simulink model "npc_plant"  (R2022a)
settings: Solver=FixedStepDiscrete  StartTime=0.0  StopTime=Inf  FixedStep=step_size  RelTol=1e-3  EnableMultiTasking=on
undefined symbols (not defined in the file): freq, L, P, step_size, vac_rms, Vdc, Vrms
libraries: spsFirstOrderFilterLib x22, spsSeriesRLCBranchLib x19, spsCurrentMeasurementLib x7, spsMosfetLib x6, spsVoltageMeasurementLib x5, spsACVoltageSourceLib x3, spsIdealSwitchLib x2, spsControlledCurrentSourceLib x1, spsDCVoltageSourceLib x1, spsGroundLib x1, spsPower3phInstantaneousLib x1, spsRMSLib x1
settings Model: DataDictionary=param.sldd  ExtModeTrigDuration=8  Creator=sgcesuser3  LastModifiedBy=sgcesuser3
settings SolverCC: AlgebraicLoopSolver=TrustRegion  AutoInsertRateTranBlk=on
settings OptimizationCC: DefaultUnderspecifiedDataType=single  EnhancedBackFolding=on  PassReuseOutputArgsAs=Individual arguments  MaxStackSize=1024  OptimizeBlockOrder=speed  DifferentSizesBufferReuse=on  OptimizationCustomize=off  DenormalBehavior=FlushToZero  EfficientTunableParamExpr=on
settings DebuggingCC: ParameterTunabilityLossMsg=error  UnconnectedInputMsg=warning  UnconnectedOutputMsg=warning  UnconnectedLineMsg=warning  SFMachineParentedDataDiag=warning
settings HardwareCC: ProdBitPerChar=16  ProdBitPerInt=16  ProdBitPerPointer=32  ProdBitPerSizeT=32  ProdBitPerPtrDiffT=32  ProdLargestAtomicInteger=Integer  ProdLargestAtomicFloat=None  ProdWordSize=16  ProdHWDeviceType=Texas Instruments->C2000
settings ModelReferenceCC: ModelReferenceNumInstancesAllowed=Single
settings SFSimCC: MATLABDynamicMemAlloc=off
settings RTWCC: SystemTargetFile=ert.tlc  HardwareBoard=TI Piccolo F280049C LaunchPad  TemplateMakefile=ert_default_tmf  Toolchain=Texas Instruments Code Composer Studio (C2000)  DLArmComputeVersion=19.05
settings CodeAppCC: ForceParamTrailComments=on  IgnoreCustomStorageClasses=off  OperatorAnnotations=on  SimulinkDataObjDesc=on  SFDataObjDesc=on  InsertBlockDesc=on
settings ERTTargetCC: CodeReplacementLibrary=TI C28x  ExtModeTransport=3  ExtModeStaticAllocSize=5000

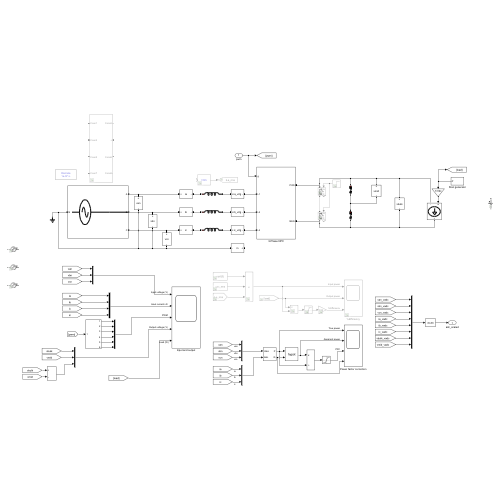
[thumbnail: Simulink's stored preview of the top-level diagram]
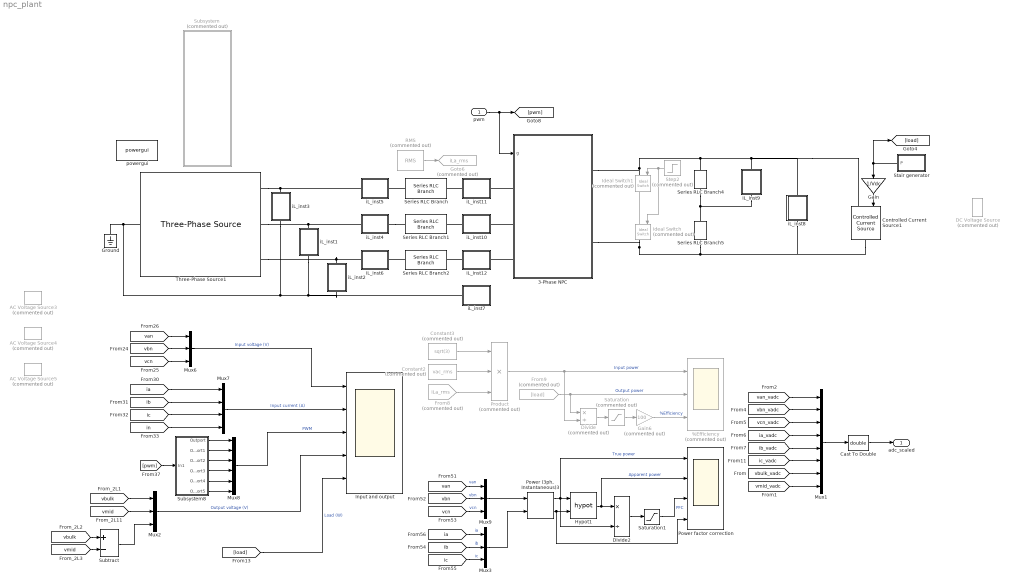
== system npc_plant ==
  pwm : Inport
  %Efficiency : Scope  Commented=on  NumInputPorts=3
  3-Phase NPC : Subsystem
  AC Voltage Source3 : spsACVoltageSourceLib/AC Voltage Source  Commented=on  Amplitude=325  Phase=0  Frequency=50  SampleTime=-1  Measurements=None  BusType=swing  Pref=10e3  Qref=0  Qmin=-inf  Qmax=+inf
  AC Voltage Source4 : spsACVoltageSourceLib/AC Voltage Source  Commented=on  Amplitude=325  Phase=0  Frequency=50  SampleTime=-1  Measurements=None  BusType=swing  Pref=10e3  Qref=0  Qmin=-inf  Qmax=+inf
  AC Voltage Source5 : spsACVoltageSourceLib/AC Voltage Source  Commented=on  Amplitude=325  Phase=0  Frequency=50  SampleTime=-1  Measurements=None  BusType=swing  Pref=10e3  Qref=0  Qmin=-inf  Qmax=+inf
  Cast To Double : DataTypeConversion  OutDataTypeStr=double  SaturateOnIntegerOverflow=off  RndMeth=Floor
  Constant2 : Constant  Commented=on  Value=vac_rms
  Constant3 : Constant  Commented=on  Value=sqrt(3)
  Controlled Current Source1 : spsControlledCurrentSourceLib/Controlled Current Source  Initialize=on  Source_Type=DC  Amplitude=0  Phase=0  Frequency=0  Measurements=None
  DC Voltage Source : spsDCVoltageSourceLib/DC Voltage Source  Commented=on  Amplitude=Vdc  Measurements=None
  Divide : Product  Commented=on  Inputs=*/
  Divide2 : Product  Inputs=*/
  From8 : From  Commented=on  GotoTag=iLa_rms  TagVisibility=global
  From9 : From  Commented=on  GotoTag=load
  Gain : Gain  Gain=1/Vdc
  Gain6 : Gain  Commented=on  Gain=100
  Goto6 : Goto  Commented=on  GotoTag=iLa_rms  TagVisibility=global
  Ground : spsGroundLib/Ground  LConnTagsString=a
  Hypot1 : Math  Operator=hypot
  Ideal Switch : spsIdealSwitchLib/Ideal Switch  Commented=on  Ron=5  Lon=0  IC=0  Rs=1e5  Cs=inf  Measurements=on
  Ideal Switch1 : spsIdealSwitchLib/Ideal Switch  Commented=on  Ron=4  Lon=0  IC=0  Rs=1e5  Cs=inf  Measurements=on
  Input and output : Scope  NumInputPorts=5
  Mux1 : Mux  Inputs=8
  Mux{2..3,6,9} (4 alike) : Mux  Inputs=3
  Mux7 : Mux
  Mux8 : Mux  Inputs=6
  "Power (3ph, Instantaneous)3" : spsPower3phInstantaneousLib/Power (3ph, Instantaneous)
  Power factor correction : Scope  NumInputPorts=4
  Product : Product  Commented=on  Inputs=3
  RMS : spsRMSLib/RMS  Commented=on  TrueRMS=on  Freq=freq  RMSInit=freq*2  Ts=step_size
  Saturation : Saturate  Commented=on  UpperLimit=1  LowerLimit=0
  Saturation1 : Saturate  UpperLimit=1  LowerLimit=0
  Series RLC Branch : spsSeriesRLCBranchLib/Series RLC Branch  LConnTagsString=__new0  RConnTagsString=__new0  BranchType=L  Resistance=1  Inductance=L  SetiL0=off  InitialCurrent=0  Capacitance=1e-6  Setx0=off  InitialVoltage=0  Measurements=None
  Series RLC Branch1 : spsSeriesRLCBranchLib/Series RLC Branch  LConnTagsString=__new0  RConnTagsString=__new0  BranchType=L  Resistance=1  Inductance=L  SetiL0=off  InitialCurrent=0  Capacitance=1e-6  Setx0=off  InitialVoltage=0  Measurements=None
  Series RLC Branch2 : spsSeriesRLCBranchLib/Series RLC Branch  LConnTagsString=__new0  RConnTagsString=__new0  BranchType=L  Resistance=1  Inductance=L  SetiL0=off  InitialCurrent=0  Capacitance=1e-6  Setx0=off  InitialVoltage=0  Measurements=None
  Series RLC Branch4 : spsSeriesRLCBranchLib/Series RLC Branch  LConnTagsString=__new0  RConnTagsString=__new0  BranchType=RC  Resistance=1e-3  Inductance=182e-6  SetiL0=off  InitialCurrent=0  Capacitance=2160e-6  Setx0=on  InitialVoltage=Vrms*sqrt(2)*sqrt(3)/2  Measurements=None
  Series RLC Branch5 : spsSeriesRLCBranchLib/Series RLC Branch  LConnTagsString=__new0  RConnTagsString=__new0  BranchType=RC  Resistance=1e-3  Inductance=182e-6  SetiL0=off  InitialCurrent=0  Capacitance=2160e-6  Setx0=on  InitialVoltage=Vrms*sqrt(2)*sqrt(3)/2  Measurements=None
  Stair generator : Subsystem
  Step2 : Step  Commented=on  Time=10  SampleTime=0
  Subsystem : Subsystem  Commented=on
  Subsystem8 : Subsystem
  Subtract : Sum  Inputs=+-
  Three-Phase Source1 : spsThreePhaseSourceLib/Three-Phase Source  InternalConnection=Yn  VoltagePhases=off  Voltage=Vrms*sqrt(3)  PhaseAngle=0  Voltage_phases=[25e3 25e3 25e3]/sqrt(3)  PhaseAngles_phases=[0 -120 +120]  Frequency=50  NonIdealSource=off  SpecifyImpedance=off  Resistance=0.8929  Inductance=16.58e-3  ShortCircuitLevel=100e6  BaseVoltage=25e3  XRratio=7  BusType=swing  Pref=10e3  Qref=0  Prefabc=[10e3, 10e3, 10e3]  Qrefabc=[0, 0, 0]  Qmin=-inf  Qmax=inf
  iL_inst1 : Subsystem
      mask Display:
      | disp('vbn')
      | port_label('Lconn',1,'+')
      | port_label('Rconn',1,'-')
  iL_inst10 : Subsystem
      mask Display:
      | disp('ib_v2g')
      | port_label('Lconn',1,'+')
      | port_label('Rconn',1,'-')
  iL_inst11 : Subsystem
      mask Display:
      | disp('ia_v2g')
      | port_label('Lconn',1,'+')
      | port_label('Rconn',1,'-')
  iL_inst12 : Subsystem
      mask Display:
      | disp('ic_v2g')
      | port_label('Lconn',1,'+')
      | port_label('Rconn',1,'-')
  iL_inst2 : Subsystem
      mask Display:
      | disp('vcn')
      | port_label('Lconn',1,'+')
      | port_label('Rconn',1,'-')
  iL_inst3 : Subsystem
      mask Display:
      | disp('van')
      | port_label('Lconn',1,'+')
      | port_label('Rconn',1,'-')
  iL_inst4 : Subsystem
      mask Display:
      | disp('ib')
      | port_label('Lconn',1,'+')
      | port_label('Rconn',1,'-')
  iL_inst5 : Subsystem
      mask Display:
      | disp('ia')
      | port_label('Lconn',1,'+')
      | port_label('Rconn',1,'-')
  iL_inst6 : Subsystem
      mask Display:
      | disp('ic')
      | port_label('Lconn',1,'+')
      | port_label('Rconn',1,'-')
  iL_inst7 : Subsystem
      mask Display:
      | disp('in')
      | port_label('Lconn',1,'+')
      | port_label('Rconn',1,'-')
  iL_inst8 : Subsystem
      mask Display:
      | disp('vbulk')
      | port_label('Lconn',1,'+')
      | port_label('Rconn',1,'-')
  iL_inst9 : Subsystem
      mask Display:
      | disp('vmid')
      | port_label('Lconn',1,'+')
      | port_label('Rconn',1,'-')
  powergui : spspowerguiLib/powergui  Priority=1  SimulationMode=Discrete  SampleTime=step_size  frequency=60  Iterations=50  frequencyindice=0  Pbase=100e6  ErrMax=1e-4  UnitsV=kV  UnitsW=MW  buscounter=0  FunctionMessages=off  echomessages=off  EnableUseOfTLC=off  CurrentSourceSwitches=off  DisableSnubberDevices=off  DisableRonSwitches=off  DisableVfSwitches=off  DisplayEquations=off  AutomaticDiscreteSolvers=off  SolverType=Tustin/Backward Euler (TBE)  Interpol=off  ExternalGateDelay=off  methode=off  Ts=100  x0status=blocks  SPID=on  SwTol=0  HookPort=off  NonlinearTolerance=1e-4  nMaxIteration=100  ContinueOnMaxIteration=off  RestoreLinks=warning  ResistiveCurrentMeasurement=off  Frange=[0:2:500]  Ylog=off  Xlog=on  ShowGrid=off  save=off  variable=ZData  structure=iLa  ZoomFFT=off  StartTime=0.12  cycles=3  DisplayStyle=2  fundamental=50  FreqAxis=on  MaxFrequency=50*41  frequencyindicesteady=1  RmsSteady=1  display=off
  adc_scaled : Outport
  wires:
  Mux1/1 -> Cast To Double/1
  Cast To Double/1 -> adc_scaled/1
  [van_vadc] -> Mux1/1
  [vbn_vadc] -> Mux1/2
  [vcn_vadc] -> Mux1/3
  [ia_vadc] -> Mux1/4
  [ic_vadc] -> Mux1/6
  [vbulk_vadc] -> Mux1/7
  [vmid_vadc] -> Mux1/8
  pwm/1 -> 3-Phase NPC/1(g), [pwm]
  Mux2/1 -> Input and output/4  "Output voltage (V)"
  [vcn] -> Mux6/3
  [van] -> Mux6/1
  [vbn] -> Mux6/2
  Mux6/1 -> Input and output/1  "Input voltage (V)"
  Mux7/1 -> Input and output/2  "Input current (A)"
  [ia] -> Mux7/1
  [ib] -> Mux7/2
  [ic] -> Mux7/3
  [pwm] -> Subsystem8/1(In1)
  Subsystem8/1(Outport) -> Mux8/1
  Subsystem8/2(Outport1) -> Mux8/2
  Subsystem8/3(Outport2) -> Mux8/3
  Subsystem8/5(Outport4) -> Mux8/5
  Subsystem8/4(Outport3) -> Mux8/4
  Subsystem8/6(Outport5) -> Mux8/6
  Mux8/1 -> Input and output/3  "PWM"
  [in] -> Mux7/4
  Step2/1 -> Ideal Switch/1, Ideal Switch1/1
  [load] -> Input and output/5  "Load (W)"
  [vmid] -> Subtract/2
  [vbulk] -> Subtract/1
  Subtract/1 -> Mux2/3
  [vmid] -> Mux2/2
  [vbulk] -> Mux2/1
  Constant3/1 -> Product/1
  Constant2/1 -> Product/2
  From8/1 -> Product/3
  Gain6/1 -> %Efficiency/3  "%Efficiency"
  Saturation/1 -> Gain6/1
  Product/1 -> Divide/2, %Efficiency/1  "Input power"
  From9/1 -> %Efficiency/2, Divide/1  "Output power"
  Divide/1 -> Saturation/1
  RMS/1 -> Goto6/1
  Saturation1/1 -> Power factor correction/3  "PFC"
  "Power (3ph, Instantaneous)3"/2 -> Power factor correction/4, Hypot1/2
  Mux9/1 -> "Power (3ph, Instantaneous)3"/1
  Mux3/1 -> "Power (3ph, Instantaneous)3"/2
  Hypot1/1 -> Divide2/1, Power factor correction/2  "Apparent power"
  "Power (3ph, Instantaneous)3"/1 -> Hypot1/1, Power factor correction/1, Divide2/2  "True power"
  Divide2/1 -> Saturation1/1
  [ic] -> Mux3/3  "ic"
  [vbn] -> Mux9/2  "vbn"
  [ib] -> Mux3/2  "ib"
  [ia] -> Mux3/1  "ia"
  [van] -> Mux9/1  "van"
  [vcn] -> Mux9/3  "vcn"
  [ib_vadc] -> Mux1/5
  Stair generator/1(P) -> Gain/1, [load]
  Gain/1 -> Controlled Current Source1/1
  connections:
  iL_inst5/LConn1 -- Three-Phase Source1/RConn1 -- iL_inst3/LConn1
  3-Phase NPC/RConn2 -- Ideal Switch/RConn1 -- Controlled Current Source1/RConn1 -- iL_inst8/RConn1 -- Series RLC Branch5/RConn1
  iL_inst4/LConn1 -- Three-Phase Source1/RConn2 -- iL_inst1/LConn1
  3-Phase NPC/LConn1 -- iL_inst11/RConn1
  iL_inst4/RConn1 -- Series RLC Branch1/LConn1
  3-Phase NPC/LConn2 -- iL_inst10/RConn1
  3-Phase NPC/LConn3 -- iL_inst12/RConn1
  Series RLC Branch/LConn1 -- iL_inst5/RConn1
  iL_inst2/LConn1 -- iL_inst6/LConn1 -- Three-Phase Source1/RConn3
  Series RLC Branch2/LConn1 -- iL_inst6/RConn1
  3-Phase NPC/RConn1 -- Ideal Switch1/LConn1 -- Controlled Current Source1/LConn1 -- iL_inst8/LConn1 -- iL_inst9/LConn1 -- Series RLC Branch4/LConn1
  iL_inst11/LConn1 -- Series RLC Branch/RConn1
  iL_inst10/LConn1 -- Series RLC Branch1/RConn1
  iL_inst12/LConn1 -- Series RLC Branch2/RConn1
  Ground/LConn1 -- Three-Phase Source1/LConn1 -- iL_inst3/RConn1 -- iL_inst1/RConn1 -- iL_inst2/RConn1 -- iL_inst7/RConn1
  Series RLC Branch5/LConn1 -- iL_inst9/RConn1 -- Series RLC Branch4/RConn1
  Ideal Switch/LConn1 -- Ideal Switch1/RConn1

== system npc_plant/3-Phase NPC ==
  g : Inport
  NPC_A : Subsystem
      settings: PortSchema="{\"entries\":[{\"content\":{\"sides\":[{\"content\":{\"connectorIds\":[\"LConn1\",\"LConn2\",\"LConn3\",\"In1\"]},\"type\":\"ConnectorPlacement.EquallySpacedRectSide\",\"uuid\":\"185b644c-5e86-499b-a0c5-6bf9ed4f6992\"},{\"content\":{\"connectorIds\":[\"RConn1\",\"RConn2\"],\"side\":\"RIGHT\"},\"type\":\"ConnectorPlacement.EquallySpacedRectSide\",\"uuid\":\"b556d60a-a111-4d52-8667-7aa86b258dfe\"},{\"content\":{\"connectorIds\":[],\"side\":\"TOP\"},\"type\":\"ConnectorPlacement.EquallySpacedRectSide\",\"uuid\":\"a387e194-6dea-4371-ac8c-2c0bb28b101b\"},{\"content\":{\"connectorIds\":[],\"side\":\"HIDDEN\"},\"type\":\"ConnectorPlacement.EquallySpacedRectSide\",\"uuid\":\"89f90e44-d209-472d-9123-cabb2f2076c2\"}]},\"type\":\"ConnectorPlacement.EquallySpacedConnector\",\"uuid\":\"47575041-459b-4ece-9f52-08593f67c377\"}],\"packageUris\":[\"http://schema.mathworks.com/mf0/Connector/R2020b\"],\"version\":\"1.0\"}"
  Series RLC Branch : spsSeriesRLCBranchLib/Series RLC Branch  LConnTagsString=__new0  RConnTagsString=__new0  BranchType=R  Resistance=1e-3  Inductance=1e-3  SetiL0=off  InitialCurrent=0  Capacitance=1e-6  Setx0=off  InitialVoltage=0  Measurements=None
  Series RLC Branch1 : spsSeriesRLCBranchLib/Series RLC Branch  LConnTagsString=__new0  RConnTagsString=__new0  BranchType=R  Resistance=1e-3  Inductance=1e-3  SetiL0=off  InitialCurrent=0  Capacitance=1e-6  Setx0=off  InitialVoltage=0  Measurements=None
  Series RLC Branch2 : spsSeriesRLCBranchLib/Series RLC Branch  LConnTagsString=__new0  RConnTagsString=__new0  BranchType=R  Resistance=1e-3  Inductance=1e-3  SetiL0=off  InitialCurrent=0  Capacitance=1e-6  Setx0=off  InitialVoltage=0  Measurements=None
  L1 : PMIOPort  Side=Left
  L2 : PMIOPort  Port=2  Side=Left
  L3 : PMIOPort  Port=3  Side=Left
  POS : PMIOPort  Port=4  Side=Right
  NEG : PMIOPort  Port=5  Side=Right
  wires:
  g/1 -> NPC_A/1(g)
  connections:
  Series RLC Branch/LConn1 -- L1/RConn1
  Series RLC Branch1/LConn1 -- L2/RConn1
  Series RLC Branch2/LConn1 -- L3/RConn1
  Series RLC Branch/RConn1 -- NPC_A/LConn1
  Series RLC Branch1/RConn1 -- NPC_A/LConn2
  Series RLC Branch2/RConn1 -- NPC_A/LConn3
  NPC_A/RConn1 -- POS/RConn1
  NEG/RConn1 -- NPC_A/RConn2

== system npc_plant/Stair generator ==
  1% : Subsystem  TreatAsAtomicUnit=on
  10% : Subsystem  TreatAsAtomicUnit=on
  100% : Subsystem  TreatAsAtomicUnit=on
  25% : Subsystem  TreatAsAtomicUnit=on
  50% : Subsystem  TreatAsAtomicUnit=on
  Digital Clock : DigitalClock  SampleTime=-1
  If : If  IfExpression=u1 > 0.7  ElseIfExpressions=u1 > 0.6, u1 > 0.5, u1 > 0.4, u1 >= 0
  Merge : Merge  Inputs=5
  P : Outport
  wires:
  Digital Clock/1 -> If/1
  If/2 -> 50%/Action
  If/4 -> 10%/Action
  If/5 -> 1%/Action
  Merge/1 -> P/1
  25%/1(Out1) -> Merge/3
  100%/1(Out1) -> Merge/1
  50%/1(Out1) -> Merge/2
  10%/1(Out1) -> Merge/4
  1%/1(Out1) -> Merge/5
  If/1 -> 100%/Action
  If/3 -> 25%/Action

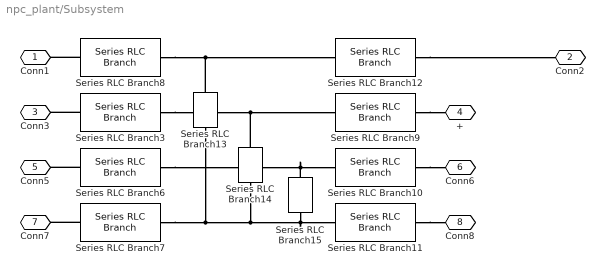
== system npc_plant/Subsystem ==
  Series RLC Branch{3,6..12} (8 alike) : spsSeriesRLCBranchLib/Series RLC Branch  LConnTagsString=__new0  RConnTagsString=__new0  BranchType=L  Resistance=1  Inductance=1.4e-3  SetiL0=off  InitialCurrent=0  Capacitance=1e-6  Setx0=off  InitialVoltage=0  Measurements=None
  Series RLC Branch13 : spsSeriesRLCBranchLib/Series RLC Branch  LConnTagsString=__new0  RConnTagsString=__new0  BranchType=C  Resistance=1  Inductance=182e-6  SetiL0=off  InitialCurrent=0  Capacitance=2.2e-6  Setx0=on  InitialVoltage=0  Measurements=None
  Series RLC Branch14 : spsSeriesRLCBranchLib/Series RLC Branch  LConnTagsString=__new0  RConnTagsString=__new0  BranchType=C  Resistance=1  Inductance=182e-6  SetiL0=off  InitialCurrent=0  Capacitance=2.2e-6  Setx0=on  InitialVoltage=0  Measurements=None
  Series RLC Branch15 : spsSeriesRLCBranchLib/Series RLC Branch  LConnTagsString=__new0  RConnTagsString=__new0  BranchType=C  Resistance=1  Inductance=182e-6  SetiL0=off  InitialCurrent=0  Capacitance=2.2e-6  Setx0=on  InitialVoltage=0  Measurements=None
  Conn1 : PMIOPort  Side=Left
  Conn2 : PMIOPort  Port=2  Side=Right
  Conn3 : PMIOPort  Port=3  Side=Left
  + : PMIOPort  Port=4  Side=Right
  Conn5 : PMIOPort  Port=5  Side=Left
  Conn6 : PMIOPort  Port=6  Side=Right
  Conn7 : PMIOPort  Port=7  Side=Left
  Conn8 : PMIOPort  Port=8  Side=Right
  connections:
  Series RLC Branch9/RConn1 -- +/RConn1
  Series RLC Branch7/RConn1 -- Series RLC Branch13/RConn1 -- Series RLC Branch14/RConn1 -- Series RLC Branch15/RConn1 -- Series RLC Branch11/LConn1
  Series RLC Branch8/RConn1 -- Series RLC Branch13/LConn1 -- Series RLC Branch12/LConn1
  Series RLC Branch6/LConn1 -- Conn5/RConn1
  Series RLC Branch7/LConn1 -- Conn7/RConn1
  Series RLC Branch6/RConn1 -- Series RLC Branch15/LConn1 -- Series RLC Branch10/LConn1
  Series RLC Branch3/RConn1 -- Series RLC Branch14/LConn1 -- Series RLC Branch9/LConn1
  Series RLC Branch12/RConn1 -- Conn2/RConn1
  Series RLC Branch11/RConn1 -- Conn8/RConn1
  Series RLC Branch10/RConn1 -- Conn6/RConn1
  Series RLC Branch3/LConn1 -- Conn3/RConn1
  Series RLC Branch8/LConn1 -- Conn1/RConn1

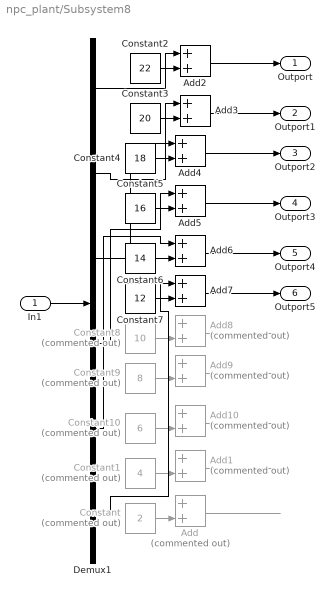
== system npc_plant/Subsystem8 ==
  In1 : Inport
  Add{,1,8..10} (5 alike) : Sum  Commented=on
  Add{2..7} (6 alike) : Sum
  Constant : Constant  Commented=on  Value=2
  Constant1 : Constant  Commented=on  Value=4
  Constant10 : Constant  Commented=on  Value=6
  Constant2 : Constant  Value=22
  Constant3 : Constant  Value=20
  Constant4 : Constant  Value=18
  Constant5 : Constant  Value=16
  Constant6 : Constant  Value=14
  Constant7 : Constant  Value=12
  Constant8 : Constant  Commented=on  Value=10
  Constant9 : Constant  Commented=on  Value=8
  Demux1 : Demux  Outputs=6
  Outport : Outport
  Outport1 : Outport  Port=2
  Outport2 : Outport  Port=3
  Outport3 : Outport  Port=4
  Outport4 : Outport  Port=5
  Outport5 : Outport  Port=6
  wires:
  ? -> Add/1
  In1/1 -> Demux1/1
  Constant/1 -> Add/2
  ? -> Add1/1
  Constant1/1 -> Add1/2
  Constant2/1 -> Add2/2
  Demux1/1 -> Add2/1
  Demux1/2 -> Add3/1
  Constant3/1 -> Add3/2
  Constant4/1 -> Add4/2
  Demux1/3 -> Add4/1
  Constant5/1 -> Add5/2
  Constant6/1 -> Add6/2
  Constant7/1 -> Add7/2
  Constant8/1 -> Add8/2
  Constant9/1 -> Add9/2
  Constant10/1 -> Add10/2
  Demux1/4 -> Add5/1
  Demux1/5 -> Add6/1
  Demux1/6 -> Add7/1
  ? -> Add8/1
  ? -> Add9/1
  ? -> Add10/1
  Add5/1 -> Outport3/1
  Add4/1 -> Outport2/1
  Add3/1 -> Outport1/1
  Add2/1 -> Outport/1
  Add6/1 -> Outport4/1
  Add7/1 -> Outport5/1
  Add8/1 -> ?
  Add9/1 -> ?
  Add10/1 -> ?
  Add1/1 -> ?
  Add/1 -> ?
  ? -> ?

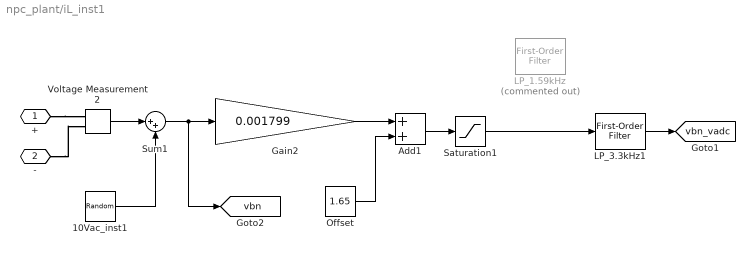
== system npc_plant/iL_inst1 ==
  10Vac_inst1 : RandomNumber  Variance=0
  Add1 : Sum
  Gain2 : Gain  Gain=0.001799
  LP_1.59kHz : spsFirstOrderFilterLib/First-Order Filter  Commented=on  FilterType=Lowpass  Tc=10e3*10e-9  Ts=step_size  Initialize=on  Vac_Init=[0, 0, 60]  Vdc_Init=0  PlotResponse=off  FreqRange="[0,  200,  1]"
  LP_3.3kHz1 : spsFirstOrderFilterLib/First-Order Filter  FilterType=Lowpass  Tc=47e-6  Ts=step_size  Initialize=on  Vac_Init=[0, 0, 60]  Vdc_Init=0  PlotResponse=off  FreqRange="[0,  200,  1]"
  Offset : Constant  Value=1.65  OutDataTypeStr=single
  Saturation1 : Saturate  UpperLimit=3.3  LowerLimit=0
  Sum1 : Sum  Inputs=|++
  Voltage Measurement2 : spsVoltageMeasurementLib/Voltage Measurement  PhasorSimulation=off  OutputType=Complex  PSBequivalent=0
  + : PMIOPort  Side=Left
  - : PMIOPort  Port=2  Side=Right
  tag scope: vbn=global, vbn_vadc=global
  wires:
  Sum1/1 -> [vbn], Gain2/1
  Offset/1 -> Add1/2
  Add1/1 -> Saturation1/1
  Gain2/1 -> Add1/1
  10Vac_inst1/1 -> Sum1/2
  Voltage Measurement2/1 -> Sum1/1
  Saturation1/1 -> LP_3.3kHz1/1
  LP_3.3kHz1/1 -> [vbn_vadc]
  connections:
  -/RConn1 -- Voltage Measurement2/LConn2
  +/RConn1 -- Voltage Measurement2/LConn1

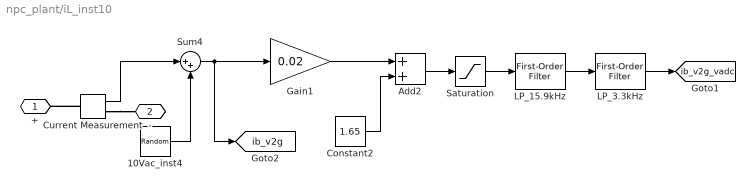
== system npc_plant/iL_inst10 ==
  10Vac_inst4 : RandomNumber  Variance=0
  Add2 : Sum
  Constant2 : Constant  Value=1.65  OutDataTypeStr=single
  Current Measurement : spsCurrentMeasurementLib/Current Measurement  PhasorSimulation=off  OutputType=Complex  PSBequivalent=0
  Gain1 : Gain  Gain=0.02
  LP_15.9kHz : spsFirstOrderFilterLib/First-Order Filter  FilterType=Lowpass  Tc=10e-6  Ts=step_size  Initialize=on  Vac_Init=[0, 0, 60]  Vdc_Init=0  PlotResponse=off  FreqRange="[0,  200,  1]"
  LP_3.3kHz : spsFirstOrderFilterLib/First-Order Filter  FilterType=Lowpass  Tc=47e-6  Ts=step_size  Initialize=on  Vac_Init=[0, 0, 60]  Vdc_Init=0  PlotResponse=off  FreqRange="[0,  200,  1]"
  Saturation : Saturate  UpperLimit=3.3  LowerLimit=0
  Sum4 : Sum  Inputs=|++
  + : PMIOPort  Side=Left
  - : PMIOPort  Port=2  Side=Right
  tag scope: ib_v2g=global, ib_v2g_vadc=global
  wires:
  10Vac_inst4/1 -> Sum4/2
  Current Measurement/1 -> Sum4/1
  Add2/1 -> Saturation/1
  Sum4/1 -> Gain1/1, [ib_v2g]
  Gain1/1 -> Add2/1
  Constant2/1 -> Add2/2
  LP_3.3kHz/1 -> [ib_v2g_vadc]
  LP_15.9kHz/1 -> LP_3.3kHz/1
  Saturation/1 -> LP_15.9kHz/1
  connections:
  Current Measurement/RConn1 -- -/RConn1
  Current Measurement/LConn1 -- +/RConn1

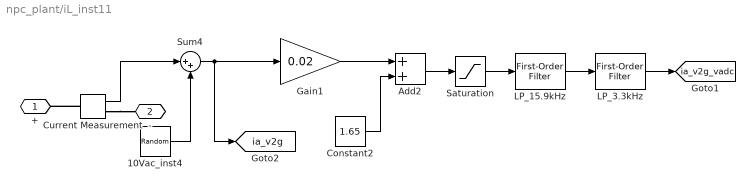
== system npc_plant/iL_inst11 ==
  10Vac_inst4 : RandomNumber  Variance=0
  Add2 : Sum
  Constant2 : Constant  Value=1.65  OutDataTypeStr=single
  Current Measurement : spsCurrentMeasurementLib/Current Measurement  PhasorSimulation=off  OutputType=Complex  PSBequivalent=0
  Gain1 : Gain  Gain=0.02
  LP_15.9kHz : spsFirstOrderFilterLib/First-Order Filter  FilterType=Lowpass  Tc=10e-6  Ts=step_size  Initialize=on  Vac_Init=[0, 0, 60]  Vdc_Init=0  PlotResponse=off  FreqRange="[0,  200,  1]"
  LP_3.3kHz : spsFirstOrderFilterLib/First-Order Filter  FilterType=Lowpass  Tc=47e-6  Ts=step_size  Initialize=on  Vac_Init=[0, 0, 60]  Vdc_Init=0  PlotResponse=off  FreqRange="[0,  200,  1]"
  Saturation : Saturate  UpperLimit=3.3  LowerLimit=0
  Sum4 : Sum  Inputs=|++
  + : PMIOPort  Side=Left
  - : PMIOPort  Port=2  Side=Right
  tag scope: ia_v2g=global, ia_v2g_vadc=global
  wires:
  Saturation/1 -> LP_15.9kHz/1
  LP_15.9kHz/1 -> LP_3.3kHz/1
  LP_3.3kHz/1 -> [ia_v2g_vadc]
  Constant2/1 -> Add2/2
  Gain1/1 -> Add2/1
  Sum4/1 -> [ia_v2g], Gain1/1
  Add2/1 -> Saturation/1
  Current Measurement/1 -> Sum4/1
  10Vac_inst4/1 -> Sum4/2
  connections:
  Current Measurement/LConn1 -- +/RConn1
  Current Measurement/RConn1 -- -/RConn1

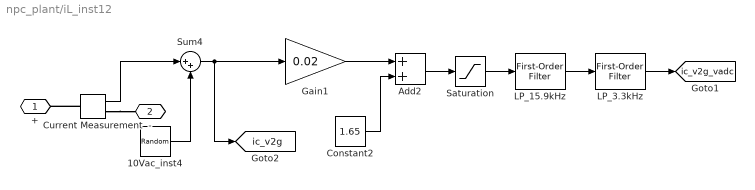
== system npc_plant/iL_inst12 ==
  10Vac_inst4 : RandomNumber  Variance=0
  Add2 : Sum
  Constant2 : Constant  Value=1.65  OutDataTypeStr=single
  Current Measurement : spsCurrentMeasurementLib/Current Measurement  PhasorSimulation=off  OutputType=Complex  PSBequivalent=0
  Gain1 : Gain  Gain=0.02
  LP_15.9kHz : spsFirstOrderFilterLib/First-Order Filter  FilterType=Lowpass  Tc=10e-6  Ts=step_size  Initialize=on  Vac_Init=[0, 0, 60]  Vdc_Init=0  PlotResponse=off  FreqRange="[0,  200,  1]"
  LP_3.3kHz : spsFirstOrderFilterLib/First-Order Filter  FilterType=Lowpass  Tc=47e-6  Ts=step_size  Initialize=on  Vac_Init=[0, 0, 60]  Vdc_Init=0  PlotResponse=off  FreqRange="[0,  200,  1]"
  Saturation : Saturate  UpperLimit=3.3  LowerLimit=0
  Sum4 : Sum  Inputs=|++
  + : PMIOPort  Side=Left
  - : PMIOPort  Port=2  Side=Right
  tag scope: ic_v2g=global, ic_v2g_vadc=global
  wires:
  10Vac_inst4/1 -> Sum4/2
  Current Measurement/1 -> Sum4/1
  Add2/1 -> Saturation/1
  Sum4/1 -> Gain1/1, [ic_v2g]
  Gain1/1 -> Add2/1
  Constant2/1 -> Add2/2
  LP_3.3kHz/1 -> [ic_v2g_vadc]
  LP_15.9kHz/1 -> LP_3.3kHz/1
  Saturation/1 -> LP_15.9kHz/1
  connections:
  Current Measurement/RConn1 -- -/RConn1
  Current Measurement/LConn1 -- +/RConn1

== system npc_plant/iL_inst2 ==
  10Vac_inst1 : RandomNumber  Variance=0
  Add1 : Sum
  Gain2 : Gain  Gain=0.001799
  LP_1.59kHz : spsFirstOrderFilterLib/First-Order Filter  Commented=on  FilterType=Lowpass  Tc=10e3*10e-9  Ts=step_size  Initialize=on  Vac_Init=[0, 0, 60]  Vdc_Init=0  PlotResponse=off  FreqRange="[0,  200,  1]"
  LP_3.3kHz1 : spsFirstOrderFilterLib/First-Order Filter  FilterType=Lowpass  Tc=47e-6  Ts=step_size  Initialize=on  Vac_Init=[0, 0, 60]  Vdc_Init=0  PlotResponse=off  FreqRange="[0,  200,  1]"
  Offset : Constant  Value=1.65  OutDataTypeStr=single
  Saturation1 : Saturate  UpperLimit=3.3  LowerLimit=0
  Sum1 : Sum  Inputs=|++
  Voltage Measurement2 : spsVoltageMeasurementLib/Voltage Measurement  PhasorSimulation=off  OutputType=Complex  PSBequivalent=0
  + : PMIOPort  Side=Left
  - : PMIOPort  Port=2  Side=Right
  tag scope: vcn=global, vcn_vadc=global
  wires:
  LP_3.3kHz1/1 -> [vcn_vadc]
  Saturation1/1 -> LP_3.3kHz1/1
  Voltage Measurement2/1 -> Sum1/1
  10Vac_inst1/1 -> Sum1/2
  Gain2/1 -> Add1/1
  Add1/1 -> Saturation1/1
  Offset/1 -> Add1/2
  Sum1/1 -> Gain2/1, [vcn]
  connections:
  +/RConn1 -- Voltage Measurement2/LConn1
  -/RConn1 -- Voltage Measurement2/LConn2

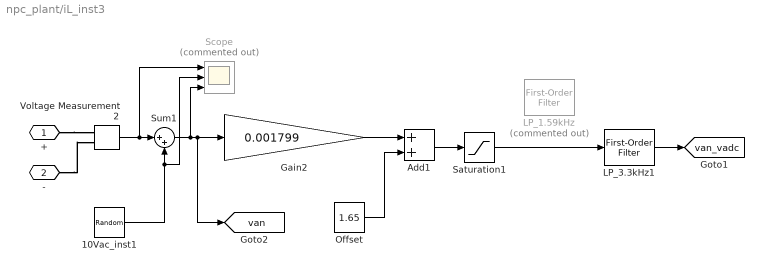
== system npc_plant/iL_inst3 ==
  10Vac_inst1 : RandomNumber  Variance=0
  Add1 : Sum
  Gain2 : Gain  Gain=0.001799
  LP_1.59kHz : spsFirstOrderFilterLib/First-Order Filter  Commented=on  FilterType=Lowpass  Tc=10e3*10e-9  Ts=step_size  Initialize=on  Vac_Init=[0, 0, 60]  Vdc_Init=0  PlotResponse=off  FreqRange="[0,  200,  1]"
  LP_3.3kHz1 : spsFirstOrderFilterLib/First-Order Filter  FilterType=Lowpass  Tc=47e-6  Ts=step_size  Initialize=on  Vac_Init=[0, 0, 60]  Vdc_Init=0  PlotResponse=off  FreqRange="[0,  200,  1]"
  Offset : Constant  Value=1.65  OutDataTypeStr=single
  Saturation1 : Saturate  UpperLimit=3.3  LowerLimit=0
  Scope : Scope  Commented=on  NumInputPorts=3
  Sum1 : Sum  Inputs=|++
  Voltage Measurement2 : spsVoltageMeasurementLib/Voltage Measurement  PhasorSimulation=off  OutputType=Complex  PSBequivalent=0
  + : PMIOPort  Side=Left
  - : PMIOPort  Port=2  Side=Right
  tag scope: van=global, van_vadc=global
  wires:
  Sum1/1 -> Scope/3, [van], Gain2/1
  Offset/1 -> Add1/2
  Add1/1 -> Saturation1/1
  Gain2/1 -> Add1/1
  10Vac_inst1/1 -> Scope/2, Sum1/2
  Voltage Measurement2/1 -> Scope/1, Sum1/1
  Saturation1/1 -> LP_3.3kHz1/1
  LP_3.3kHz1/1 -> [van_vadc]
  connections:
  -/RConn1 -- Voltage Measurement2/LConn2
  +/RConn1 -- Voltage Measurement2/LConn1

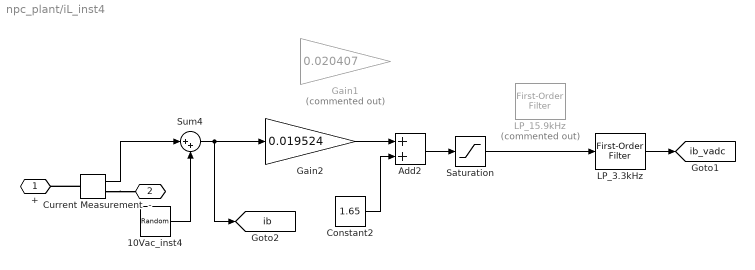
== system npc_plant/iL_inst4 ==
  10Vac_inst4 : RandomNumber  Variance=0
  Add2 : Sum
  Constant2 : Constant  Value=1.65  OutDataTypeStr=single
  Current Measurement : spsCurrentMeasurementLib/Current Measurement  PhasorSimulation=off  OutputType=Complex  PSBequivalent=0
  Gain1 : Gain  Commented=on  Gain=0.020407
  Gain2 : Gain  Gain=0.019524
  LP_15.9kHz : spsFirstOrderFilterLib/First-Order Filter  Commented=on  FilterType=Lowpass  Tc=10e-6  Ts=step_size  Initialize=on  Vac_Init=[0, 0, 60]  Vdc_Init=0  PlotResponse=off  FreqRange="[0,  200,  1]"
  LP_3.3kHz : spsFirstOrderFilterLib/First-Order Filter  FilterType=Lowpass  Tc=47e-6  Ts=step_size  Initialize=on  Vac_Init=[0, 0, 60]  Vdc_Init=0  PlotResponse=off  FreqRange="[0,  200,  1]"
  Saturation : Saturate  UpperLimit=3.3  LowerLimit=0
  Sum4 : Sum  Inputs=|++
  + : PMIOPort  Side=Left
  - : PMIOPort  Port=2  Side=Right
  tag scope: ib=global, ib_vadc=global
  wires:
  Saturation/1 -> LP_3.3kHz/1
  LP_3.3kHz/1 -> [ib_vadc]
  Constant2/1 -> Add2/2
  Gain2/1 -> Add2/1
  Sum4/1 -> Gain2/1, [ib]
  Add2/1 -> Saturation/1
  Current Measurement/1 -> Sum4/1
  10Vac_inst4/1 -> Sum4/2
  connections:
  Current Measurement/LConn1 -- +/RConn1
  Current Measurement/RConn1 -- -/RConn1

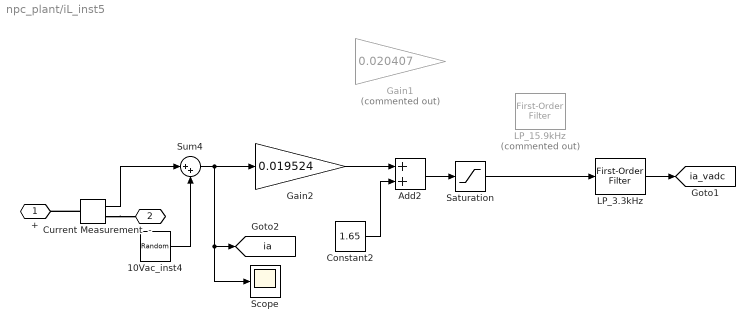
== system npc_plant/iL_inst5 ==
  10Vac_inst4 : RandomNumber  Variance=0
  Add2 : Sum
  Constant2 : Constant  Value=1.65  OutDataTypeStr=single
  Current Measurement : spsCurrentMeasurementLib/Current Measurement  PhasorSimulation=off  OutputType=Complex  PSBequivalent=0
  Gain1 : Gain  Commented=on  Gain=0.020407
  Gain2 : Gain  Gain=0.019524
  LP_15.9kHz : spsFirstOrderFilterLib/First-Order Filter  Commented=on  FilterType=Lowpass  Tc=10e-6  Ts=step_size  Initialize=on  Vac_Init=[0, 0, 60]  Vdc_Init=0  PlotResponse=off  FreqRange="[0,  200,  1]"
  LP_3.3kHz : spsFirstOrderFilterLib/First-Order Filter  FilterType=Lowpass  Tc=47e-6  Ts=step_size  Initialize=on  Vac_Init=[0, 0, 60]  Vdc_Init=0  PlotResponse=off  FreqRange="[0,  200,  1]"
  Saturation : Saturate  UpperLimit=3.3  LowerLimit=0
  Scope : Scope
  Sum4 : Sum  Inputs=|++
  + : PMIOPort  Side=Left
  - : PMIOPort  Port=2  Side=Right
  tag scope: ia=global, ia_vadc=global
  wires:
  10Vac_inst4/1 -> Sum4/2
  Current Measurement/1 -> Sum4/1
  Add2/1 -> Saturation/1
  Sum4/1 -> Gain2/1, Scope/1, [ia]
  Gain2/1 -> Add2/1
  Constant2/1 -> Add2/2
  LP_3.3kHz/1 -> [ia_vadc]
  Saturation/1 -> LP_3.3kHz/1
  connections:
  Current Measurement/RConn1 -- -/RConn1
  Current Measurement/LConn1 -- +/RConn1

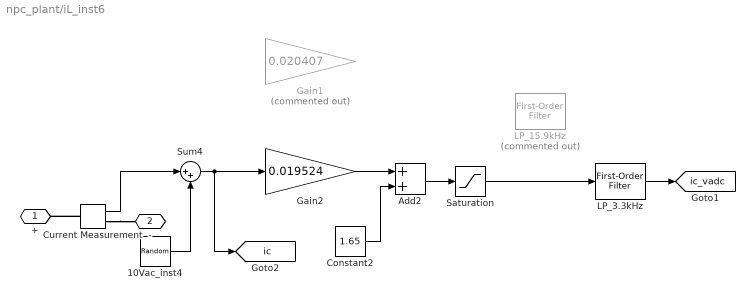
== system npc_plant/iL_inst6 ==
  10Vac_inst4 : RandomNumber  Variance=0
  Add2 : Sum
  Constant2 : Constant  Value=1.65  OutDataTypeStr=single
  Current Measurement : spsCurrentMeasurementLib/Current Measurement  PhasorSimulation=off  OutputType=Complex  PSBequivalent=0
  Gain1 : Gain  Commented=on  Gain=0.020407
  Gain2 : Gain  Gain=0.019524
  LP_15.9kHz : spsFirstOrderFilterLib/First-Order Filter  Commented=on  FilterType=Lowpass  Tc=10e-6  Ts=step_size  Initialize=on  Vac_Init=[0, 0, 60]  Vdc_Init=0  PlotResponse=off  FreqRange="[0,  200,  1]"
  LP_3.3kHz : spsFirstOrderFilterLib/First-Order Filter  FilterType=Lowpass  Tc=47e-6  Ts=step_size  Initialize=on  Vac_Init=[0, 0, 60]  Vdc_Init=0  PlotResponse=off  FreqRange="[0,  200,  1]"
  Saturation : Saturate  UpperLimit=3.3  LowerLimit=0
  Sum4 : Sum  Inputs=|++
  + : PMIOPort  Side=Left
  - : PMIOPort  Port=2  Side=Right
  tag scope: ic=global, ic_vadc=global
  wires:
  Saturation/1 -> LP_3.3kHz/1
  LP_3.3kHz/1 -> [ic_vadc]
  Constant2/1 -> Add2/2
  Gain2/1 -> Add2/1
  Sum4/1 -> Gain2/1, [ic]
  Add2/1 -> Saturation/1
  Current Measurement/1 -> Sum4/1
  10Vac_inst4/1 -> Sum4/2
  connections:
  Current Measurement/LConn1 -- +/RConn1
  Current Measurement/RConn1 -- -/RConn1

== system npc_plant/iL_inst7 ==
  Current Measurement : spsCurrentMeasurementLib/Current Measurement  PhasorSimulation=off  OutputType=Complex  PSBequivalent=0
  + : PMIOPort  Side=Left
  - : PMIOPort  Port=2  Side=Right
  tag scope: in=global
  wires:
  Current Measurement/1 -> [in]
  connections:
  Current Measurement/RConn1 -- -/RConn1
  Current Measurement/LConn1 -- +/RConn1

== system npc_plant/iL_inst8 ==
  10Vac_inst4 : RandomNumber  Variance=0
  Gain1 : Gain  Gain=0.0036102
  LP_128Hz : spsFirstOrderFilterLib/First-Order Filter  Commented=on  FilterType=Lowpass  Tc=0.001236443  Ts=step_size  Initialize=on  Vac_Init=[0, 0, 60]  Vdc_Init=0  PlotResponse=off  FreqRange="[0,  200,  1]"
  LP_15.9kHz_1 : spsFirstOrderFilterLib/First-Order Filter  FilterType=Lowpass  Tc=10e-6  Ts=step_size  Initialize=on  Vac_Init=[0, 0, 60]  Vdc_Init=0  PlotResponse=off  FreqRange="[0,  200,  1]"
  Saturation : Saturate  UpperLimit=3.3  LowerLimit=0
  Sum4 : Sum  Inputs=|++
  Voltage Measurement2 : spsVoltageMeasurementLib/Voltage Measurement  PhasorSimulation=off  OutputType=Complex  PSBequivalent=0
  + : PMIOPort  Side=Left
  - : PMIOPort  Port=2  Side=Right
  tag scope: vbulk=global, vbulk_vadc=global
  wires:
  LP_15.9kHz_1/1 -> [vbulk_vadc]
  Sum4/1 -> Gain1/1, [vbulk]
  Saturation/1 -> LP_15.9kHz_1/1
  Gain1/1 -> Saturation/1
  Voltage Measurement2/1 -> Sum4/1
  10Vac_inst4/1 -> Sum4/2
  connections:
  Voltage Measurement2/LConn1 -- +/RConn1
  -/RConn1 -- Voltage Measurement2/LConn2

== system npc_plant/iL_inst9 ==
  10Vac_inst4 : RandomNumber  Variance=0
  Gain1 : Gain  Gain=0.0064528
  LP_128Hz_2 : spsFirstOrderFilterLib/First-Order Filter  FilterType=Lowpass  Tc=0.001236443  Ts=step_size  Initialize=on  Vac_Init=[0, 0, 60]  Vdc_Init=0  PlotResponse=off  FreqRange="[0,  200,  1]"
  LP_15.9kHz_3 : spsFirstOrderFilterLib/First-Order Filter  FilterType=Lowpass  Tc=10e-6  Ts=step_size  Initialize=on  Vac_Init=[0, 0, 60]  Vdc_Init=0  PlotResponse=off  FreqRange="[0,  200,  1]"
  Saturation : Saturate  UpperLimit=3.3  LowerLimit=0
  Sum4 : Sum  Inputs=|++
  Voltage Measurement2 : spsVoltageMeasurementLib/Voltage Measurement  PhasorSimulation=off  OutputType=Complex  PSBequivalent=0
  + : PMIOPort  Side=Left
  - : PMIOPort  Port=2  Side=Right
  tag scope: vmid=global, vmid_vadc=global
  wires:
  Sum4/1 -> Gain1/1, [vmid]
  LP_15.9kHz_3/1 -> [vmid_vadc]
  Saturation/1 -> LP_15.9kHz_3/1
  Gain1/1 -> Saturation/1
  Voltage Measurement2/1 -> Sum4/1
  10Vac_inst4/1 -> Sum4/2
  connections:
  -/RConn1 -- Voltage Measurement2/LConn2
  Voltage Measurement2/LConn1 -- +/RConn1

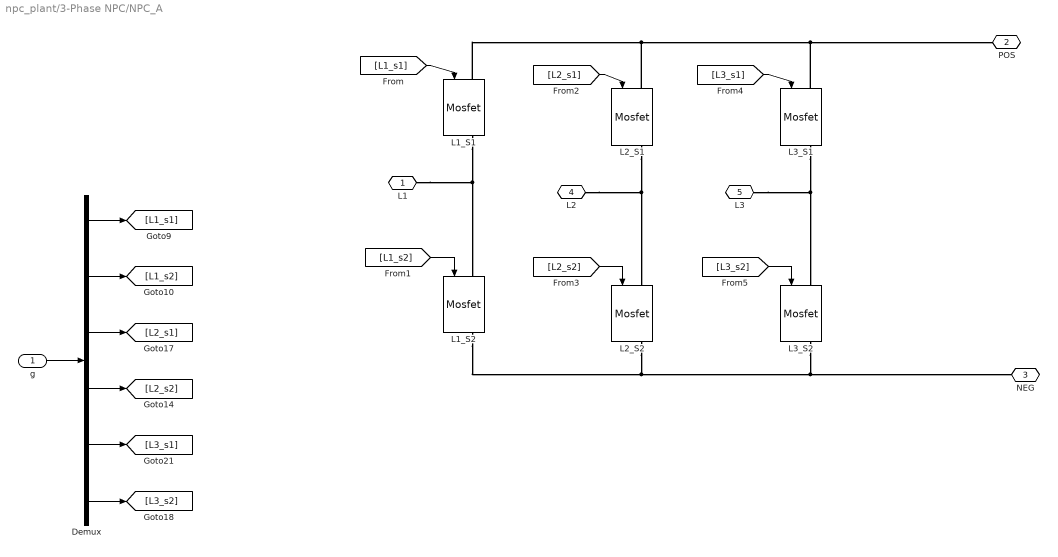
== system npc_plant/3-Phase NPC/NPC_A ==
  g : Inport
  Demux : Demux  Outputs=6
  L1_S1 : spsMosfetLib/Mosfet  Ron=0.1  Lon=0  Rd=0.01  Vfd=0  IC=0  Rs=1e5  Cs=inf  Measurements=on
  L1_S2 : spsMosfetLib/Mosfet  Ron=0.1  Lon=0  Rd=0.01  Vfd=0  IC=0  Rs=1e5  Cs=inf  Measurements=on
  L2_S1 : spsMosfetLib/Mosfet  Ron=0.1  Lon=0  Rd=0.01  Vfd=0  IC=0  Rs=1e5  Cs=inf  Measurements=on
  L2_S2 : spsMosfetLib/Mosfet  Ron=0.1  Lon=0  Rd=0.01  Vfd=0  IC=0  Rs=1e5  Cs=inf  Measurements=on
  L3_S1 : spsMosfetLib/Mosfet  Ron=0.1  Lon=0  Rd=0.01  Vfd=0  IC=0  Rs=1e5  Cs=inf  Measurements=on
  L3_S2 : spsMosfetLib/Mosfet  Ron=0.1  Lon=0  Rd=0.01  Vfd=0  IC=0  Rs=1e5  Cs=inf  Measurements=on
  L1 : PMIOPort  Side=Left
  POS : PMIOPort  Port=2  Side=Right
  NEG : PMIOPort  Port=3  Side=Right
  L2 : PMIOPort  Port=4  Side=Left
  L3 : PMIOPort  Port=5  Side=Left
  wires:
  [L1_s2] -> L1_S2/1
  [L1_s1] -> L1_S1/1
  [L2_s1] -> L2_S1/1
  [L2_s2] -> L2_S2/1
  [L3_s2] -> L3_S2/1
  [L3_s1] -> L3_S1/1
  Demux/1 -> [L1_s1]
  g/1 -> Demux/1
  Demux/4 -> [L2_s2]
  Demux/2 -> [L1_s2]
  Demux/3 -> [L2_s1]
  Demux/6 -> [L3_s2]
  Demux/5 -> [L3_s1]
  connections:
  L1_S1/RConn1 -- L1/RConn1 -- L1_S2/LConn1
  L1_S1/LConn1 -- L2_S1/LConn1 -- POS/RConn1 -- L3_S1/LConn1
  L1_S2/RConn1 -- L2_S2/RConn1 -- L3_S2/RConn1 -- NEG/RConn1
  L2/RConn1 -- L2_S1/RConn1 -- L2_S2/LConn1
  L3_S1/RConn1 -- L3/RConn1 -- L3_S2/LConn1

== system npc_plant/Stair generator/1% ==
  Action Port : ActionPort  ActionPortLabel=elseif( u1 >= 0)
  Constant : Constant  Value=0.01*P
  Out1 : Outport
  wires:
  Constant/1 -> Out1/1

== system npc_plant/Stair generator/10% ==
  Action Port : ActionPort  ActionPortLabel=elseif( u1 > 0.4)
  Constant : Constant  Value=0.1*P
  Out1 : Outport
  wires:
  Constant/1 -> Out1/1

== system npc_plant/Stair generator/100% ==
  Action Port : ActionPort  ActionPortLabel=if(u1 > 0.7)
  Constant : Constant  Value=1*P
  Out1 : Outport
  wires:
  Constant/1 -> Out1/1

== system npc_plant/Stair generator/25% ==
  Action Port : ActionPort  ActionPortLabel=elseif( u1 > 0.5)
  Constant : Constant  Value=0.25*P
  Out1 : Outport
  wires:
  Constant/1 -> Out1/1

== system npc_plant/Stair generator/50% ==
  Action Port : ActionPort  ActionPortLabel=elseif(u1 > 0.6)
  Constant : Constant  Value=0.5*P
  Out1 : Outport
  wires:
  Constant/1 -> Out1/1
